simulink model "sar_model"  (R2020b)
settings: Solver=VariableStepAuto  StartTime=0.0  StopTime=4.0  FixedStep=0.001  RelTol=1e-3
InitFcn:
  | stop_time_as_str = get_param(gcs, 'StopTime');
  | flightTime = str2double(stop_time_as_str);
model workspace: external: MAT-File /Users/tomoffat/Documents/final_year_coursework/fyp/blender/sar_consts.mat (data not in the file)
values from neighbouring files (symbols this model uses):
  aperture = 4    [sar_consts.mat]    (also in sar_script_ref.m)
  c = physconst('LightSpeed')    [omegak.m]    (also in sar_consts.mat = 299792458; sar_script_ref.m)
  fc = 4000000000    [sar_consts.mat]    (also in sar_script_ref.m)
  speed = 400    [sar_consts.mat]    (also in sar_script_ref.m = 100)
  tpd = 3e-06    [sar_consts.mat]    (also in sar_script_ref.m)
undefined symbols (not defined in the file or in its folder): aperture2gain, phased, physconst
libraries: phasedenvlib x5, phasedtxrxlib x4, vrlib x2, phasedwavlib x1, dspsigops x1
settings Model: SimulationMode=accelerator  Creator=tomoffat  LastModifiedBy=tomoffat

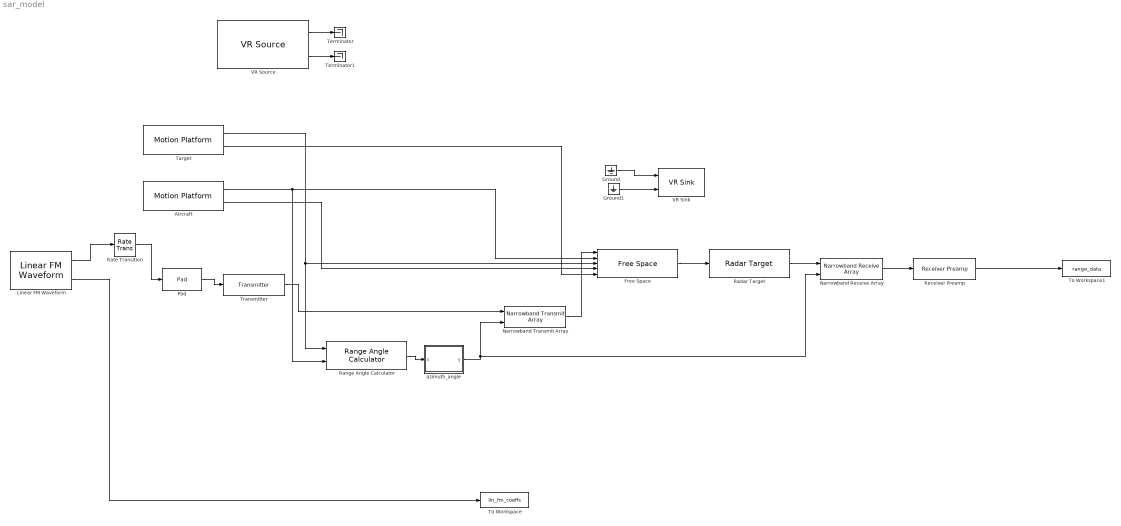
== system sar_model ==
  Aircraft : phasedenvlib/Motion Platform  MotionModel=Velocity  InitialPosition=[ 500; 1000; -1000 ]  InitialVelocity=[ 0; 0; 0 ]  VelocitySource=Property  Velocity=[0;0;speed]  AccelerationSource=Property  Acceleration=[0;0;0]  CustomTrajectory=[ 0, 0, 0, 0, 0, 0, 0; 1, 0, 0, 0, 0, 0, 0 ]  ScanMode=None  InitialScanAngle=0  AzimuthSpan=[ -60, 60 ]  AzimuthScanRate=10  InitialOrientationAxes=eye( 3 )  OrientationAxesOutputPort=off  ElapsedTimeSource=Auto  SampleRateFromInputCheckbox=on  SampleRate=1e6  SimulateUsing=Interpreted execution
      settings: SourceProductBaseCode=AR
  Free Space : phasedenvlib/Free Space  PropagationSpeed=physconst( 'LightSpeed' )  OperatingFrequency=fc  TwoWayPropagation=on  SampleRateFromInputCheckbox=off  SampleRate=1.2E8  MaximumDistanceSource=Property  MaximumDistance=10e3  MaximumNumInputSamplesSource=Auto  MaximumNumInputSamples=1000  SimulateUsing=Interpreted execution
      settings: SourceProductBaseCode=AR
  Ground : Ground
  Ground1 : Ground
  Linear FM Waveform : phasedwavlib/Linear FM Waveform  SampleRate=1.2E8  DurationSpecification=Pulse width  PulseWidth=tpd  DutyCycle=0.5  PRF=prf  PRFSelectionInputPort=off  SimulationTimeSource=Derive from waveform parameters  SweepBandwidth=bw  SweepDirection=Up  SweepInterval=Positive  Envelope=Rectangular  FrequencyOffsetSource=Property  FrequencyOffset=0  OutputFormat=Pulses  NumSamples=100  NumPulses=4001  PRFOutputPort=off  CoefficientsOutputPort=on  SimulateUsing=Interpreted execution
      settings: SourceProductBaseCode=AR
  Narrowband Receive Array : phasedtxrxlib/Narrowband Receive Array  PropagationSpeed=physconst( 'LightSpeed' )  OperatingFrequency=fc  Wavefront=Plane  SensorGainMeasure=dB  Polarization=None  WeightsInputPort=off  SimulateUsing=Interpreted execution  Sensor=phased.CosineAntennaElement('FrequencyRange',[1e6 6e9])
      settings: SourceProductBaseCode=AR
  Narrowband Transmit Array : phasedtxrxlib/Narrowband Transmit Array  PropagationSpeed=physconst( 'LightSpeed' )  OperatingFrequency=fc  CombineRadiatedSignals=on  SensorGainMeasure=dB  Polarization=None  WeightsInputPort=off  SimulateUsing=Interpreted execution  Sensor=phased.CosineAntennaElement('FrequencyRange',[1e9 6e9])
      settings: SourceProductBaseCode=AR
  Pad : dspsigops/Pad  padAlong=Specified dimensions  dimsToPad=1  valSrc=Specify via dialog  padVal=0  spec=Output size  padNumOutRowsSpecMethod=User-specified  numOutRows=1  padNumOutColsSpecMethod=User-specified  numOutCols=1  isVarDimsMode=off  padBeginning=0  padEnd=0  outSizeMode=User-specified  outSize=2002  padSigAt=End  trunc_flag=None  roundingMode=Floor  overflowMode=off  truncOrWrapMode=Truncate  wrap_flag=None
      settings: SourceProductBaseCode=DS
  Radar Target : phasedenvlib/Radar Target  EnablePolarization=off  Mode=Monostatic  MeanRCSSource=Property  ScatteringMatrixSource=Property  MeanRCS=20  ScatteringMatrix=eye( 2 )  Model=Nonfluctuating  PropagationSpeed=physconst( 'LightSpeed' )  OperatingFrequency=fc  SeedSource=Auto  Seed=0  SimulateUsing=Interpreted execution
      settings: SourceProductBaseCode=AR
  Range Angle Calculator : phasedenvlib/Range Angle Calculator  Model=Free space  ReferencePositionSource=Input port  ReferencePosition=[ 0; 0; 0 ]  ReferenceAxesSource=Property  ReferenceAxes=eye( 3 )  Output=Angle  SimulateUsing=Interpreted execution
      settings: SourceProductBaseCode=AR
  Rate Transition : RateTransition  Deterministic=off
  Receiver Preamp : phasedtxrxlib/Receiver Preamp  Gain=20  LossFactor=0  NoiseMethod=Noise temperature  NoiseFigure=30  ReferenceTemperature=290  SampleRateFromInputCheckbox=off  SampleRate=1.2E8  NoisePower=0  EnableInputPort=off  PhaseNoiseInputPort=off  SeedSource=Auto  Seed=0  SimulateUsing=Interpreted execution
      settings: SourceProductBaseCode=AR
  Target : phasedenvlib/Motion Platform  MotionModel=Velocity  InitialPosition=targetpos  InitialVelocity=[ 0; 0; 0 ]  VelocitySource=Property  Velocity=[0;0;0]  AccelerationSource=Property  Acceleration=[0;0;0]  CustomTrajectory=[ 0, 0, 0, 0, 0, 0, 0; 1, 0, 0, 0, 0, 0, 0 ]  ScanMode=None  InitialScanAngle=0  AzimuthSpan=[ -60, 60 ]  AzimuthScanRate=10  InitialOrientationAxes=eye( 3 )  OrientationAxesOutputPort=off  ElapsedTimeSource=Auto  SampleRateFromInputCheckbox=on  SampleRate=1e6  SimulateUsing=Interpreted execution
      settings: SourceProductBaseCode=AR
  Terminator : Terminator
  Terminator1 : Terminator
  To Workspace : ToWorkspace  VariableName=lin_fm_coeffs  SampleTime=-1
      settings: Save2DSignal=2-D array (concatenate along first dimension)
  To Workspace1 : ToWorkspace  VariableName=range_data  SampleTime=-1
      settings: Save2DSignal=2-D array (concatenate along first dimension)
  Transmitter : phasedtxrxlib/Transmitter  PeakPower=50e3  Gain=aperture2gain(aperture,c/fc)  LossFactor=0  InUseOutputPort=off  CoherentOnTransmit=on  PhaseNoiseOutputPort=off  SeedSource=Auto  Seed=0  SimulateUsing=Interpreted execution
      settings: SourceProductBaseCode=AR
  VR Sink : vrlib/VR Sink  InstantiateOnLoad=on  SampleTime=0.1  ViewEnable=on  RemoteChange=off  RemoteView=off  FieldsWritten=shape_terminal.translation.3.1.1.double#shape_plane.translation.3.1.1.double  WorldFileName=3d_test_model.x3d  WorldDescription=Testing a 3D model  AutoView=on  VideoDimensions=[]  AllowVariableSize=off  FigureProperties="{'Position', 'Name', 'Viewpoint', 'CameraBound', 'CameraDirection', 'CameraPosition', 'CameraUpVector', 'ZoomFactor', 'Antialiasing', 'Headlight', 'Lighting', 'NavPanel', 'Sound', 'StatusBar', 'Stereo3D', 'Stereo3DCameraOffset', 'Stereo3DHIT', 'ToolBar', 'Textures', 'Transparency', 'Triad', 'Wireframe', 'NavZones', 'NavMode', 'NavSpeed', 'CaptureFileFormat', 'CaptureFileName', 'Record2DCompressMethod', 'Record2DCompressQuality', 'Record2D', 'Record2DFileName', 'Record2DFPS'; [1.7310000000000000e+03  -2.2200000000000000e+02   5.7600000000000000e+02   3.5000000000000000e+02], 'Testing a 3D model', 'Overview for editing', 'on', [0.0000000000000000e+00   0.0000000000000000e+00  -1.0000000000000000e+00], [0.0000000000000000e+00   0.0000000000000000e+00   0.0000000000000000e+00], [0.0000000000000000e+00   1.0000000000000000e+00   0.0000000000000000e+00], [1.0000000000000000e+00], 'on', 'on', 'on', 'halfbar', 'on', 'on', 'off', [1.0000000149011612e-01], [0.0000000000000000e+00], 'on', 'on', 'on', 'none', 'off', 'off', 'fly', 'normal', 'tif', '%f_anim_%n.tif', 'auto', [7.5000000000000000e+01], 'off', '%f_anim_%n.avi', 'auto'}"
  VR Source : vrlib/VR Source  InstantiateOnLoad=on  SampleTime=0.1  ViewEnable=on  RemoteChange=off  RemoteView=off  FieldsRead=shape_terminal.scale.1.3.1.double#Building_Round_IFS_Coord.point.209.3.1.double  WorldFileName=3d_test_model.x3d  WorldDescription=Testing a 3D model  AutoView=off  VideoDimensions=[]  AllowVariableSize=off
      settings: SourceProductBaseCode=SL
  azimuth_angle : MATLAB Function  TreatAsAtomicUnit=on
  wires:
  Aircraft/1 -> Free Space/2, Range Angle Calculator/2
  Target/1 -> Free Space/3, Range Angle Calculator/1
  Aircraft/2 -> Free Space/4
  Target/2 -> Free Space/5
  Free Space/1 -> Radar Target/1
  Transmitter/1 -> Narrowband Transmit Array/1
  Narrowband Transmit Array/1 -> Free Space/1
  Range Angle Calculator/1 -> azimuth_angle/1(u)
  azimuth_angle/1(y) -> Narrowband Transmit Array/2, Narrowband Receive Array/2
  Radar Target/1 -> Narrowband Receive Array/1
  Narrowband Receive Array/1 -> Receiver Preamp/1
  Linear FM Waveform/2 -> To Workspace/1
  VR Source/1 -> Terminator/1
  VR Source/2 -> Terminator1/1
  Pad/1 -> Transmitter/1
  Linear FM Waveform/1 -> Rate Transition/1
  Rate Transition/1 -> Pad/1
  Ground/1 -> VR Sink/1
  Ground1/1 -> VR Sink/2
  Receiver Preamp/1 -> To Workspace1/1

== matlab function sar_model/azimuth_angle ==
  data: u input; y output; targetpos parameter
function y = azimuth_angle(u, targetpos)
refangle = zeros(1, size(targetpos,2));
u(1,:) = refangle;
y = u;
